simulink library "lib_Convection_DittusBoelter"  (R2015a)
settings: Solver=ode45  StartTime=0.0  StopTime=10.0  RelTol=1e-3
libraries: simulink x3
settings Model: Creator=jlkratz  LastModifiedBy=jlkratz

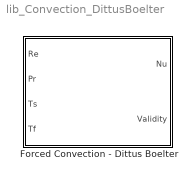
== system lib_Convection_DittusBoelter ==
  Forced Convection - Dittus Boelter : Subsystem  mask(TSAT: Dittus-Boelter Block){}
      mask help:
      | The block approximates the local Nusselt number for fully developed turbulent flow in a smooth circular tube using the Dittus-Boelter equation. For tubes with different shaped cross-sections this correlation can be used a first approximation with the hydraulic diameter of the tube used in place of the tube diameter. The equation has some dependence on whether the tube is being heated or cooled and hence the need for temperature inputs for the surface of the tube (Ts) and mean temperature of the fluid (Tf). All properties should be evaluated at the mean fluid temperature Tf. This correlation has the following restrictions:
      |
      | 0.6 <= Pr <= 160
      | Re >= 10000
      | L/D >= 10 (L/D = entrance length / diameter) <-- fully developed
      |
      | This correlation is a good approxiamtion for uniform surface temperature and heat flux conditions. If there are large variations in the temperature and thus properties then the Sieder-Tate correlation may be a better approximation.
      mask Help: web(which('Convection_TSAT_DittusBoelter.html'),'-helpbrowser')

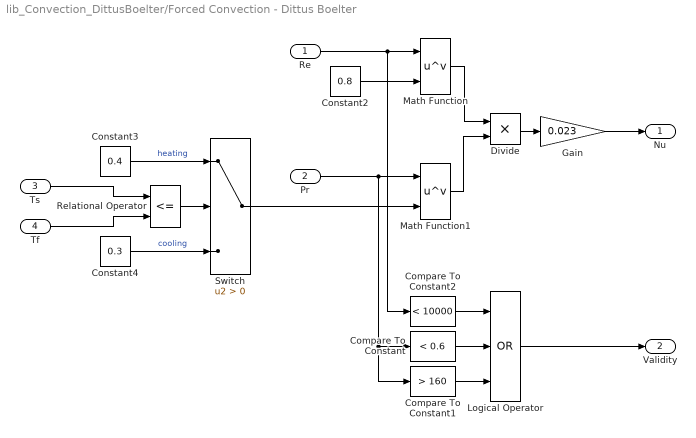
== system lib_Convection_DittusBoelter/Forced Convection - Dittus Boelter ==
  Re : Inport
  Pr : Inport  Port=2
  Ts : Inport  Port=3
  Tf : Inport  Port=4
  Compare To Constant : simulink/Logic and Bit Operations/Compare To Constant  relop=<  const=0.6  OutDataTypeStr=boolean
  Compare To Constant1 : simulink/Logic and Bit Operations/Compare To Constant  relop=>  const=160  OutDataTypeStr=boolean
  Compare To Constant2 : simulink/Logic and Bit Operations/Compare To Constant  relop=<  const=10000  OutDataTypeStr=boolean
  Constant2 : Constant  Value=0.8
  Constant3 : Constant  Value=0.4
  Constant4 : Constant  Value=0.3
  Divide : Product  Inputs=**
  Gain : Gain  Gain=0.023
  Logical Operator : Logic  Operator=OR  Inputs=3  AllPortsSameDT=off  OutDataTypeStr=boolean
  Math Function : Math  Operator=pow  SaturateOnIntegerOverflow=on
  Math Function1 : Math  Operator=pow  SaturateOnIntegerOverflow=on
  Relational Operator : RelationalOperator  Operator=<=  OutDataTypeStr=boolean
  Switch : Switch  Criteria=u2 > Threshold
  Nu : Outport
  Validity : Outport  Port=2
  wires:
  Tf/1 -> Relational Operator/2
  Switch/1 -> Math Function1/2
  Ts/1 -> Relational Operator/1
  Gain/1 -> Nu/1
  Pr/1 -> Math Function1/1, Compare To Constant/1, Compare To Constant1/1
  Constant3/1 -> Switch/1  "heating"
  Constant4/1 -> Switch/3  "cooling"
  Math Function/1 -> Divide/1
  Divide/1 -> Gain/1
  Re/1 -> Math Function/1, Compare To Constant2/1
  Compare To Constant1/1 -> Logical Operator/3
  Logical Operator/1 -> Validity/1
  Compare To Constant/1 -> Logical Operator/2
  Compare To Constant2/1 -> Logical Operator/1
  Relational Operator/1 -> Switch/2
  Math Function1/1 -> Divide/2
  Constant2/1 -> Math Function/2
